simulink model "Problem_1"  (R2020b)
settings: Solver=VariableStepAuto  StartTime=0.0  StopTime=1  RelTol=1e-3
model workspace (MAT data in the model file):
  B = Simulink.Parameter
  B.Value = 50
  B.DataType = 'auto'
  B.Dimensions = [1 1]
  K1 = Simulink.Parameter
  K1.Value = 50
  K1.DataType = 'auto'
  K1.Dimensions = [1 1]
  K12 = Simulink.Parameter
  K12.Value = 1000
  K12.DataType = 'auto'
  K12.Dimensions = [1 1]
  M1 = Simulink.Parameter
  M1.Value = 100
  M1.DataType = 'auto'
  M1.Dimensions = [1 1]
  M2 = Simulink.Parameter
  M2.Value = 50
  M2.DataType = 'auto'
  M2.Dimensions = [1 1]
settings Model: Creator=Yeshwanth  LastModifiedBy=Yeshwanth

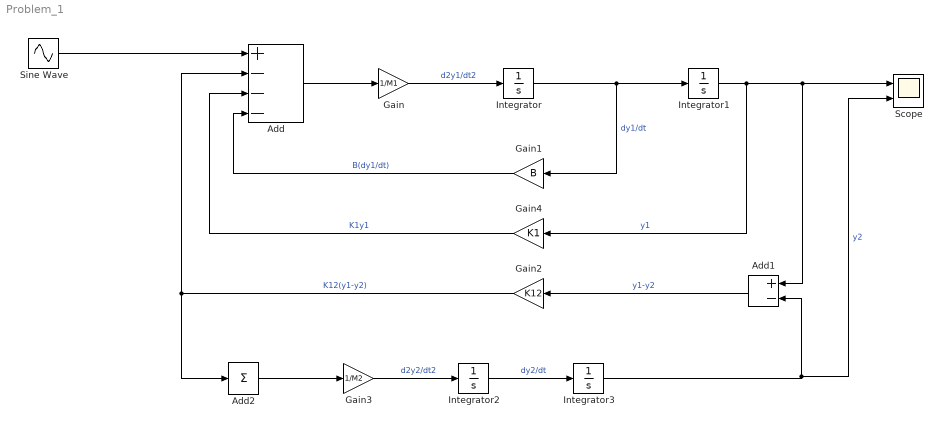
== system Problem_1 ==
  Add : Sum  Inputs=+---
  Add1 : Sum  Inputs=+-
  Add2 : Sum  Inputs=+
  Gain : Gain  Gain=1/M1
  Gain1 : Gain  Gain=B
  Gain2 : Gain  Gain=K12
  Gain3 : Gain  Gain=1/M2
  Gain4 : Gain  Gain=K1
  Integrator{,1..3} (4 alike) : Integrator
  Scope : Scope  NumInputPorts=2
  Sine Wave : Sin  Amplitude=2  Frequency=10  SampleTime=0
  wires:
  Add/1 -> Gain/1
  Gain/1 -> Integrator/1  "d2y1/dt2"
  Integrator/1 -> Gain1/1, Integrator1/1  "dy1/dt"
  Gain1/1 -> Add/4  "B(dy1/dt)"
  Integrator1/1 -> Gain4/1, Scope/1, Add1/1  "y1"
  Gain4/1 -> Add/3  "K1y1"
  Integrator2/1 -> Integrator3/1  "dy2/dt"
  Gain3/1 -> Integrator2/1  "d2y2/dt2"
  Integrator3/1 -> Scope/2, Add1/2  "y2"
  Add1/1 -> Gain2/1  "y1-y2"
  Sine Wave/1 -> Add/1
  Add2/1 -> Gain3/1
  Gain2/1 -> Add2/1, Add/2  "K12(y1-y2)"
